simulink model "Ex_Feb_2014_2"  (R2022b)
settings: Solver=VariableStepAuto  StartTime=0.0  StopTime=150  RelTol=1e-3
settings Model: Creator=rrilo  LastModifiedBy=rrilo

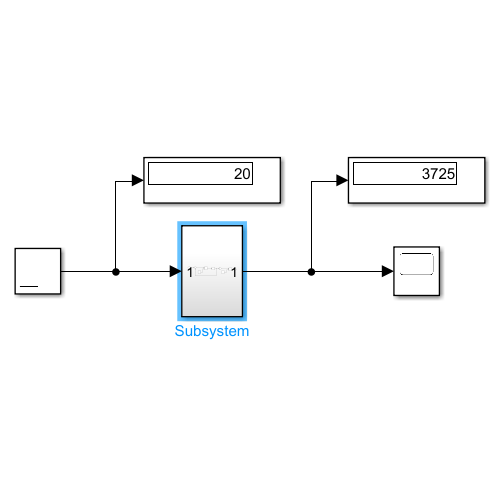
[thumbnail: Simulink's stored preview of the top-level diagram]
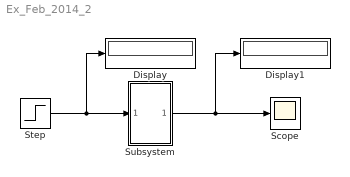
== system Ex_Feb_2014_2 ==
  Display : Display
  Display1 : Display
  Scope : Scope
  Step : Step  After=20  SampleTime=0
  Subsystem : Subsystem
  wires:
  Subsystem/1(Out1) -> Display1/1, Scope/1
  Step/1 -> Display/1, Subsystem/1(In1)

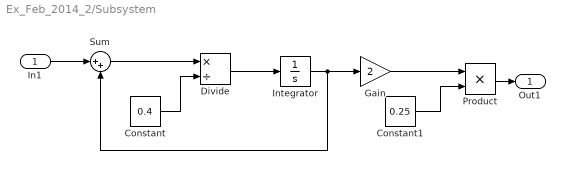
== system Ex_Feb_2014_2/Subsystem ==
  In1 : Inport
  Constant : Constant  Value=0.4
  Constant1 : Constant  Value=0.25
  Divide : Product  Inputs=*/
  Gain : Gain  Gain=2
  Integrator : Integrator  IgnoreLimit=on
  Product : Product
  Sum : Sum  Inputs=|++
  Out1 : Outport
  wires:
  Product/1 -> Out1/1
  Constant1/1 -> Product/2
  Gain/1 -> Product/1
  Integrator/1 -> Sum/2, Gain/1
  Sum/1 -> Divide/1
  Divide/1 -> Integrator/1
  In1/1 -> Sum/1
  Constant/1 -> Divide/2
